simulink model "AE_315_W2_RL_circuit_current"  (R2022b)
settings: Solver=VariableStepAuto  StartTime=0.0  StopTime=10.0  RelTol=1e-3
settings Model: Creator=SoftLaptop  LastModifiedBy=SoftLaptop

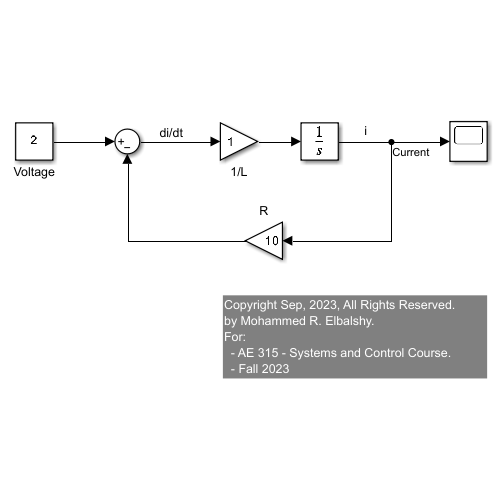
[thumbnail: Simulink's stored preview of the top-level diagram]
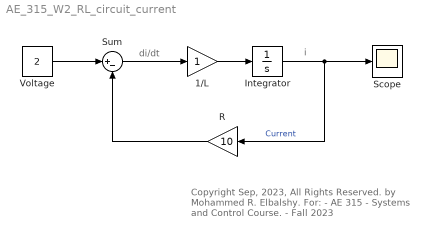
== system AE_315_W2_RL_circuit_current ==
  note: di/dt
  note: i
  note: Copyright Sep, 2023, All Rights Reserved.
      | by Mohammed R. Elbalshy.
      | For:
      | - AE 315 - Systems and Control Course.
      | - Fall 2023
  1/L : Gain
  Integrator : Integrator
  R : Gain  Gain=10
  Scope : Scope
  Sum : Sum  Inputs=|+-
  Voltage : Constant  Value=2
  wires:
  Voltage/1 -> Sum/1
  R/1 -> Sum/2
  Sum/1 -> 1/L/1
  Integrator/1 -> Scope/1, R/1  "Current"
  1/L/1 -> Integrator/1
